simulink model "Encoding_Encryption_Model"  (R2024a)
settings: Solver=VariableStepAuto  StartTime=0.0  StopTime=10.0  RelTol=1e-3
libraries: commdigbbndpm3 x2, simulink x2
settings Model: Creator=adcli  LastModifiedBy=adcli
settings RTWCC: GPUComputeCapability=3.5

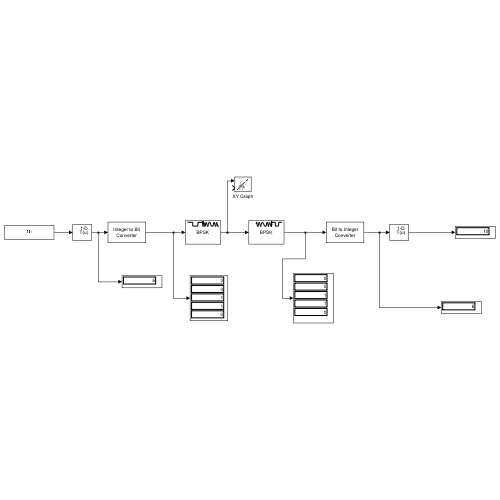
[thumbnail: Simulink's stored preview of the top-level diagram]
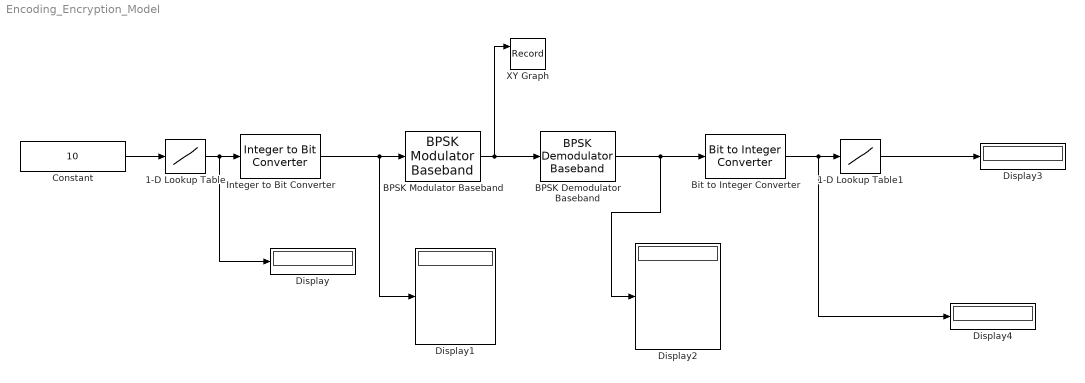
== system Encoding_Encryption_Model ==
  1-D Lookup Table : Lookup_n-D  NumberOfTableDimensions=1  BreakpointsForDimension1=[0:15]  Table=[2, 15, 8, 3, 7, 11, 0, 4, 9, 10, 6, 13, 5, 12, 14, 1]  InternalRulePriority=Speed  RndMeth=Simplest
  1-D Lookup Table1 : Lookup_n-D  NumberOfTableDimensions=1  BreakpointsForDimension1=[0:15]  Table=[6, 15, 0, 3, 7, 12, 10, 4, 2, 8, 9, 5, 13, 11, 14, 1]  InternalRulePriority=Speed  RndMeth=Simplest
  BPSK Demodulator Baseband : commdigbbndpm3/BPSK Demodulator Baseband  DecType=Hard decision  VarSource=Dialog  Variance=1  Ph=0  outDtype=Inherit via internal rule  derotateFactorWordLen=16  derotateFactorDataTypeStr=Inherit: Same word length as input  derotateFactorLastDataTypeStr=Inherit: Same word length as input
  BPSK Modulator Baseband : commdigbbndpm3/BPSK Modulator Baseband  Ph=0  outDtype=double  outWordLen=16  outUDDataType=sfix(16)  outFracLenMode=Best precision  outFracLen=15  outDataTypeStr=double  outLastDataTypeStr=double
  Bit to Integer Converter : simulink/Logic and Bit Operations/Bit to Integer Converter  nbits=5  bitOrder=MSB first  signedOutputValues=Unsigned  outDtype=Inherit via internal rule  outDtypeSigned=Inherit via internal rule
  Constant : Constant  Value=10
  Display{,1..4} (5 alike) : Display
  Integer to Bit Converter : simulink/Logic and Bit Operations/Integer to Bit Converter  nbits=5  signedInputValues=Unsigned  bitOrder=MSB first  outDtype=Inherit via internal rule
  XY Graph : Record  FileSettingsInternal="{\"entries\":[{\"content\":{\"excelSettings\":{\"content\":{},\"type\":\"Streamout.ExcelSettings\"}},\"type\":\"Streamout.FileSettingStorage\",\"uuid\":\"\"}],\"packageUris\":[\"http:\\/\\/schema.mathworks.com\\/mf0\\/streamout_blocks\\/R2020a\"],\"version\":\"1.0\"}"  Layout=[1 1]  SignalsInternal="{\"entries\":[{\"content\":{\"signals\":[{\"content\":{\"blockPath\":[],\"dimensions\":[5],\"domain\":\"\",\"hasChildren\":true,\"isComplex\":true,\"lineColor\":\"#7e2f8e\",\"lineWidth\":2,\"port\":1,\"sid\":[\"\"],\"signalID\":1,\"signalName\":\"BPSK\\nModulator\\nBaseband\"},\"type\":\"RecordBlkView.Signal\",\"uuid\":\"\"},{\"content\":{\"blockPath\":[],\"channel\":[1],\"dimensions\":[5],\"domain\":\"\",\"hasChildren\":true,\"isComplex\":true,\"lineColor\":\"#77ac30\",\"lineWidth\":2,\"parentID\":1,\"port\":1,\"sid\":[\"\"],\"signalID\":2,\"signalName\":\"BPSK\\nModulator\\nBaseband\"},\"type\":\"RecordBlkView.Signal\",\"uuid\":\"\"},{\"content\":{\"blockPath\":[],\"dimensions\":[5],\"domain\":\"\",\"isComplex\":true,\"lineColor\":\"#4dbeee\",\"lineWidth\":2,\"parentID\":2,\"port\":1,\"sid\":[\"\"],\"signalID\":3,\"signalName\":\"BPSK\\nModulator\\nBaseband\"},\"type\":\"RecordBlkView.Signal\",\"uuid\":\"\"},{\"content\":{\"blockPath\":[],\"dimensions\":[5],\"domain\":\"\",\"imagPart\":true,\"isComplex\":true,\"lineColor\":\"#a2142f\",\"lineWidth\":2,\"parentID\":2,\"port\":1,\"sid\":[\"\"],\"signalID\":4,\"signalName\":\"BPSK\\nModulator\\nBaseband\"},\"type\":\"RecordBlkView.Signal\",\"uuid\":\"\"},{\"content\":{\"blockPath\":[],\"dimensions\":[1],\"domain\":\"\",\"lineColor\":\"#139fff\",\"lineWidth\":2,\"port\":2,\"sid\":[\"\"],\"signalID\":5},\"type\":\"RecordBlkView.Signal\",\"uuid\":\"\"}]},\"type\":\"RecordBlkView.InputSignals\",\"uuid\":\"\"}],\"packageUris\":[\"http:\\/\\/schema.mathworks.com\\/mf0\\/streamout_blocks\\/R2020a\"],\"version\":\"1.0\"}"  VisualizationBindings="{\"xyplotplugin\":{\"info\":[{\"series\":[],\"subplotID\":1}]}}"  CompatibilityTag=XY
  wires:
  BPSK Modulator Baseband/1 -> BPSK Demodulator Baseband/1, XY Graph/1
  BPSK Demodulator Baseband/1 -> Bit to Integer Converter/1, Display2/1
  Integer to Bit Converter/1 -> Display1/1, BPSK Modulator Baseband/1
  Constant/1 -> 1-D Lookup Table/1
  1-D Lookup Table/1 -> Display/1, Integer to Bit Converter/1
  Bit to Integer Converter/1 -> 1-D Lookup Table1/1, Display4/1
  1-D Lookup Table1/1 -> Display3/1
